simulink model "SEA_model_ConstInput"  (Simulink 7.2)
settings: Solver=ode45  StartTime=0.0  StopTime=100  RelTol=1e-3
values from neighbouring files (symbols this model uses):
  b = 0.0575    [TSC150918ProvaMatlab.m]
  d = 2.5185    [TSC150918ProvaMatlab.m]
  g = 9.81    [TSC150918ProvaMatlab.m]
  j = 0.2156    [TSC150918ProvaMatlab.m]
  k = 200    [TSC150918ProvaMatlab.m]
  l = 0.5    [TSC150918ProvaMatlab.m]
  m = 0.15    [TSC150918ProvaMatlab.m]
  taue = 0.2    [TSC150918ProvaMatlab.m]
  X0 = Xe + Dx0    [TSC150918ProvaMatlab.m]
settings Model: Creator=lbiagiotti  LastModifiedBy=lbiagiotti

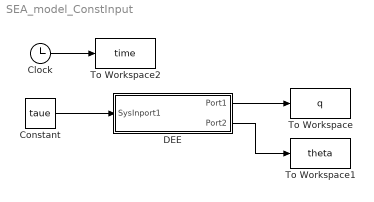
== system SEA_model_ConstInput ==
  Clock : Clock
      settings: Decimation=10
  Constant : Constant  Value=taue  OutDataType=sfix(16)  OutScaling=2^0
  DEE : Subsystem
      settings: OpenFcn=diffeqed
      mask Type: Differential Equation Editor (DEE)
      mask Display: disp('Differential Equation\n Editor')
  To Workspace : ToWorkspace  VariableName=q  SampleTime=-1  SaveFormat=Array
  To Workspace1 : ToWorkspace  VariableName=theta  SampleTime=-1  SaveFormat=Array
  To Workspace2 : ToWorkspace  VariableName=time  SampleTime=-1  SaveFormat=Array
  wires:
  Constant/1 -> DEE/1(SysInport1)
  DEE/1(Port1) -> To Workspace/1
  DEE/2(Port2) -> To Workspace1/1
  Clock/1 -> To Workspace2/1

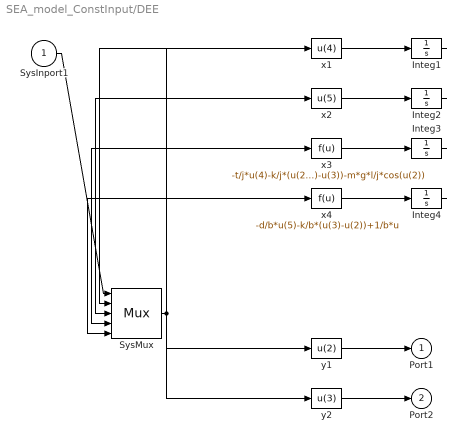
== system SEA_model_ConstInput/DEE ==
  SysInport1 : Inport
  Integ1 : Integrator  InitialCondition=X0(1)
  Integ2 : Integrator  InitialCondition=X0(2)
  Integ3 : Integrator  InitialCondition=X0(3)
  Integ4 : Integrator  InitialCondition=X0(4)
  SysMux : Mux  Inputs=5
  x1 : Fcn  Expr=u(4)
  x2 : Fcn  Expr=u(5)
  x3 : Fcn  Expr=-t/j*u(4)-k/j*(u(2)-u(3))-m*g*l/j*cos(u(2))
  x4 : Fcn  Expr=-d/b*u(5)-k/b*(u(3)-u(2))+1/b*u
  y1 : Fcn  Expr=u(2)
  y2 : Fcn  Expr=u(3)
  Port1 : Outport
  Port2 : Outport  Port=2
  wires:
  SysInport1/1 -> SysMux/1
  SysMux/1 -> x1/1, x2/1, x3/1, x4/1, y1/1, y2/1
  x1/1 -> Integ1/1
  Integ1/1 -> SysMux/2
  x2/1 -> Integ2/1
  Integ2/1 -> SysMux/3
  x3/1 -> Integ3/1
  Integ3/1 -> SysMux/4
  x4/1 -> Integ4/1
  Integ4/1 -> SysMux/5
  y1/1 -> Port1/1
  y2/1 -> Port2/1
